simulink model "assignment1"  (R2020b)
settings: Solver=VariableStepAuto  StartTime=0.0  StopTime=10.0  RelTol=1e-3
settings Model: Creator=Sudhanshu  LastModifiedBy=Sudhanshu

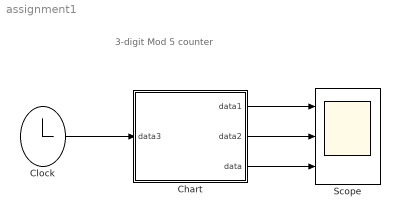
== system assignment1 ==
  note: 3-digit Mod 5 counter
  Chart : Stateflow chart  TreatAsAtomicUnit=on
  Clock : Clock
  Scope : Scope  NumInputPorts=3
  wires:
  Chart/3(data) -> Scope/3
  Chart/1(data1) -> Scope/1
  Chart/2(data2) -> Scope/2
  Clock/1 -> Chart/1(data3)

== stateflow chart assignment1/Chart ==
  state State1
    en:
    a=0;
    b=0;
    c=0;
  state State2
    en:
    c=0;
    b=0;
    a=1;
  state State3
    en:
    c=0;
    b=1;
    a=0;
  state State4
    en:
    c=0;
    b=1;
    a=1;
  state State5
    en:
    c=1;
    b=0;
    a=0;
  (default) -> State1
  State5 -> State1 : {c==1 && b==0 && a==0}
  State1 -> State2 : {c==0 && b==0 && a==0}
  State2 -> State3 : {c==0 && b==0 && a==1}
  State3 -> State4 : {c==0 && b==1 && a==0}
  State4 -> State5 : {c==0 && b==1 && a==1}
  data: data1 output; data2 output; data output; data3 input
